simulink model "robot_model_open"  (R2018b)
settings: Solver=ode15s  StartTime=0.0  StopTime=26  RelTol=1e-3  EnableMultiTasking=on
libraries: simulink_extras x4
settings Model: Creator=Akos  LastModifiedBy=akos
settings DataIOCC: LimitDataPoints=on  SaveFormat=Array
settings OptimizationCC: LifeSpan=inf
settings DebuggingCC: SFUnexpectedBacktrackingDiag=warning  SFNoUnconditionalDefaultTransitionDiag=warning  SFExecutionAtInitializationDiag=none
settings HardwareCC: ProdBitPerPointer=32  ProdBitPerSizeT=32  ProdBitPerPtrDiffT=32  ProdLargestAtomicFloat=None  ProdIntDivRoundTo=Undefined  ProdEndianess=Unspecified  ProdWordSize=32  ProdHWDeviceType=32-bit Generic
settings ModelReferenceCC: PropagateSignalLabelsOutOfModel=off
settings SFSimCC: SimUseLocalCustomCode=off
settings RTWCC: RTWUseLocalCustomCode=off
settings CodeAppCC: StateflowObjectComments=on
settings GRTTargetCC: TargetLangStandard=C89/C90 (ANSI)  GeneratePreprocessorConditionals=Disable all
settings ConfigComp: CovMetricSettings=dw  CovHtmlReporting=on  CovSaveCumulativeToWorkspaceVar=on  CovSaveSingleToWorkspaceVar=on  CovExternalEMLEnable=off

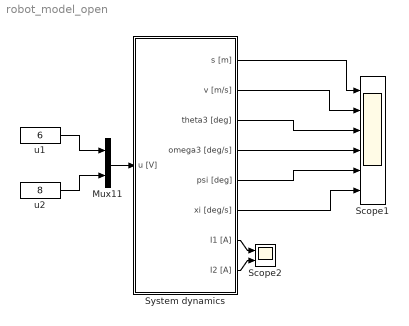
== system robot_model_open ==
  Mux11 : Mux  Inputs=2
  Scope1 : Scope  NumInputPorts=6
  Scope2 : Scope  NumInputPorts=2
  System dynamics : Subsystem
  u1 : Constant  Value=6
  u2 : Constant  Value=8
  wires:
  System dynamics/7(I1 [A]) -> Scope2/1
  System dynamics/8(I2 [A]) -> Scope2/2
  Mux11/1 -> System dynamics/1(u [V])
  System dynamics/1(s [m]) -> Scope1/1
  System dynamics/2(v [m/s]) -> Scope1/2
  System dynamics/3(theta3 [deg]) -> Scope1/3
  System dynamics/4(omega3 [deg/s]) -> Scope1/4
  System dynamics/5(psi [deg]) -> Scope1/5
  System dynamics/6(xi [deg/s]) -> Scope1/6
  u1/1 -> Mux11/1
  u2/1 -> Mux11/2

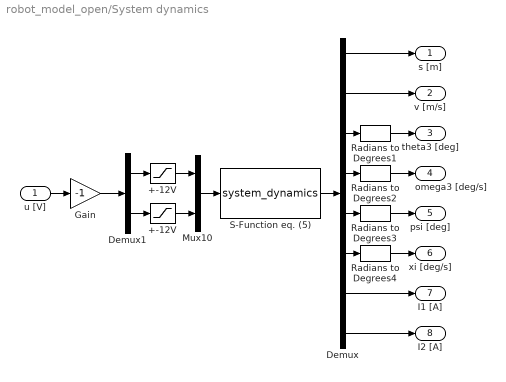
== system robot_model_open/System dynamics ==
  u [V] : Inport
  +-12V : Saturate  UpperLimit=12  LowerLimit=-12
  "+-12V " : Saturate  UpperLimit=12  LowerLimit=-12
  Demux : Demux  Outputs=8
  Demux1 : Demux  Outputs=2
  Gain : Gain  Gain=-1
  Mux10 : Mux  Inputs=2
  Radians to Degrees{1..4} (4 alike) : simulink_extras/Transformations/Radians to Degrees
  S-Function eq. (5) : S-Function  FunctionName=system_dynamics  SFunctionDeploymentMode=off  EnableBusSupport=off
  s [m] : Outport
  v [m/s] : Outport  Port=2
  theta3 [deg] : Outport  Port=3
  omega3 [deg/s] : Outport  Port=4
  psi [deg] : Outport  Port=5
  xi [deg/s] : Outport  Port=6
  I1 [A] : Outport  Port=7
  I2 [A] : Outport  Port=8
  wires:
  Demux/2 -> v [m/s]/1
  Demux/1 -> s [m]/1
  Demux/3 -> Radians to Degrees1/1
  Demux/7 -> I1 [A]/1
  Demux/8 -> I2 [A]/1
  Mux10/1 -> S-Function eq. (5)/1
  S-Function eq. (5)/1 -> Demux/1
  Demux/6 -> Radians to Degrees4/1
  Demux/5 -> Radians to Degrees3/1
  Demux/4 -> Radians to Degrees2/1
  +-12V/1 -> Mux10/1
  "+-12V "/1 -> Mux10/2
  Radians to Degrees1/1 -> theta3 [deg]/1
  Radians to Degrees2/1 -> omega3 [deg/s]/1
  Radians to Degrees3/1 -> psi [deg]/1
  Radians to Degrees4/1 -> xi [deg/s]/1
  u [V]/1 -> Gain/1
  Demux1/1 -> +-12V/1
  Demux1/2 -> "+-12V "/1
  Gain/1 -> Demux1/1
